simulink model "SXQCIVI"  (R2021b)
settings: Solver=FixedStepDiscrete  StartTime=0.0  StopTime=inf  FixedStep=0.005  RelTol=1e-3
undefined symbols (not defined in the file): calss, EngineTWT_Enginerunhours, EngineTWT_EnginerunhoursState, NVM_CFG_ENG_TYPE, NVM_HFV_Enginerunhours, REV_EngineSpeed, REV_EngineSpeedState, rte_set_uint32_val, rte_set_uint8_val, RXSIG_EngHrRev_Total_engine_hours, SIG_CLASS_COMTX, SIG_CLASS_NVM, SIG_CLASS_NVM_CFG, SIG_CLASS_SWC, TXSIG_EngHrRev_EGR_Total_engine_hours, TXSIG_HOURS_EGR_EngineTotalHoursofOperation, type, value
settings Model: Creator=huangyanlong  LastModifiedBy=huangyanlong
settings OptimizationCC: DefaultParameterBehavior=Inlined  EnhancedBackFolding=on  PassReuseOutputArgsAs=Individual arguments  ZeroExternalMemoryAtStartup=off  ZeroInternalMemoryAtStartup=off  OptimizeBlockOrder=speed  DifferentSizesBufferReuse=on  OptimizationCustomize=off  EfficientTunableParamExpr=on
settings DebuggingCC: ParameterTunabilityLossMsg=error
settings SFSimCC: MATLABDynamicMemAlloc=off
settings RTWCC: Description=Embedded Coder  SystemTargetFile=ert.tlc  GenCodeOnly=on  TemplateMakefile=ert_default_tmf  GenerateReport=on  IncludeHyperlinkInReport=on  LaunchReport=on  GenerateTraceInfo=on  GenerateTraceReport=on  GenerateTraceReportSl=on  GenerateTraceReportSf=on  GenerateTraceReportEml=on  GenerateWebview=on  GenerateCodeMetricsReport=on  GenerateCodeReplacementReport=on
settings CodeAppCC: ForceParamTrailComments=on  IgnoreCustomStorageClasses=off  OperatorAnnotations=on  SimulinkDataObjDesc=on  SFDataObjDesc=on  InsertBlockDesc=on
settings ERTTargetCC: TargetLangStandard=C99 (ISO)  GenerateSampleERTMain=on  InlinedParameterPlacement=NonHierarchical  ERTCustomFileTemplate=example_file_process.tlc

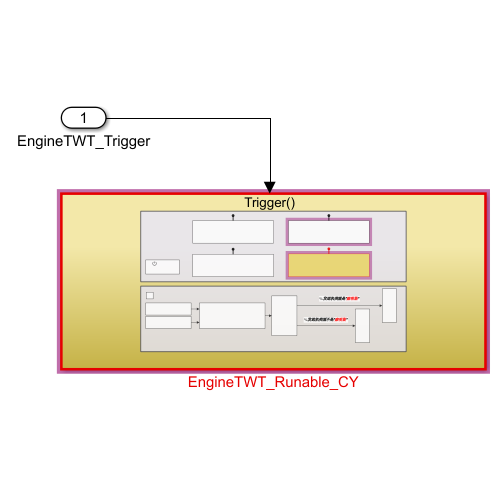
[thumbnail: Simulink's stored preview of the top-level diagram]
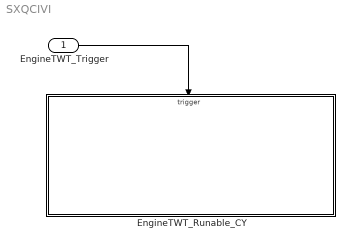
== system SXQCIVI ==
  EngineTWT_Trigger : Inport  SampleTime=0.01  OutputFunctionCall=on
  EngineTWT_Runable_CY : Subsystem
  wires:
  EngineTWT_Trigger/1 -> EngineTWT_Runable_CY/Trigger

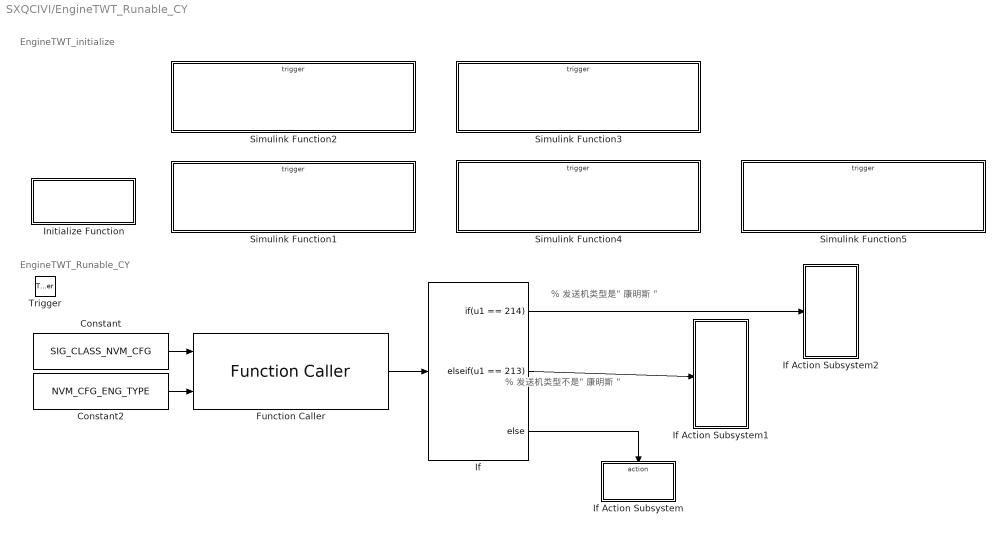
== system SXQCIVI/EngineTWT_Runable_CY ==
  note: % 发送机类型是" 康明斯 "
  note: EngineTWT_Runable_CY
  note: EngineTWT_initialize
  note: % 发送机类型不是" 康明斯 "
  Trigger : TriggerPort  TriggerType=function-call  VariantControl=(inherit)  SampleTimeType=periodic  SampleTime=0.01  PortDimensions=1
  Constant : Constant  Value=SIG_CLASS_NVM_CFG  OutDataTypeStr=int8
  Constant2 : Constant  Value=NVM_CFG_ENG_TYPE  OutDataTypeStr=int8
  Function Caller : FunctionCaller  FunctionPrototype=ret = rte_get_uint16_val(calss,type)  InputArgumentSpecifications=int8(1),int8(1)  OutputArgumentSpecifications=int16(1)
  If : If  IfExpression=u1 == 214  ElseIfExpressions=u1 == 213
  If Action Subsystem : Subsystem  TreatAsAtomicUnit=on
  If Action Subsystem1 : Subsystem  TreatAsAtomicUnit=on
  If Action Subsystem2 : Subsystem  TreatAsAtomicUnit=on
  Initialize Function : Subsystem  TreatAsAtomicUnit=on
  Simulink Function1 : Subsystem  TreatAsAtomicUnit=on
  Simulink Function2 : Subsystem  TreatAsAtomicUnit=on
  Simulink Function3 : Subsystem  TreatAsAtomicUnit=on
  Simulink Function4 : Subsystem  TreatAsAtomicUnit=on
  Simulink Function5 : Subsystem  TreatAsAtomicUnit=on
  wires:
  Constant/1 -> Function Caller/1
  Constant2/1 -> Function Caller/2
  Function Caller/1 -> If/1
  If/1 -> If Action Subsystem2/Action
  If/2 -> If Action Subsystem1/Action
  If/3 -> If Action Subsystem/Action

== system SXQCIVI/EngineTWT_Runable_CY/If Action Subsystem ==
  Action Port : ActionPort  ActionPortLabel=else

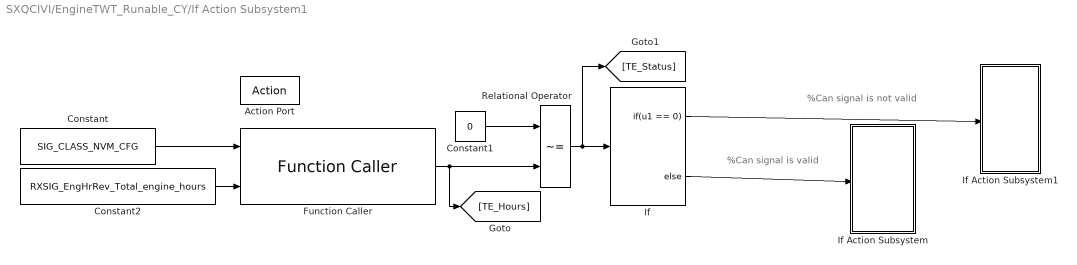
== system SXQCIVI/EngineTWT_Runable_CY/If Action Subsystem1 ==
  note: %Can signal is not valid
  note: %Can signal is valid
  Action Port : ActionPort  ActionPortLabel=elseif(u1 == 213)
  Constant : Constant  Value=SIG_CLASS_NVM_CFG  OutDataTypeStr=int8
  Constant1 : Constant  Value=0
  Constant2 : Constant  Value=RXSIG_EngHrRev_Total_engine_hours  OutDataTypeStr=int8
  Function Caller : FunctionCaller  FunctionPrototype=ret = rte_get_uint32_val(calss,type)  InputArgumentSpecifications=int8(1),int8(1)  OutputArgumentSpecifications=int32(1)
  If : If  IfExpression=u1 == 0
  If Action Subsystem : Subsystem  TreatAsAtomicUnit=on
  If Action Subsystem1 : Subsystem  TreatAsAtomicUnit=on
  Relational Operator : RelationalOperator  Operator=~=  OutDataTypeStr=boolean  RndMeth=Simplest
  wires:
  Relational Operator/1 -> [TE_Status], If/1
  Function Caller/1 -> [TE_Hours], Relational Operator/2
  Constant2/1 -> Function Caller/2
  Constant/1 -> Function Caller/1
  Constant1/1 -> Relational Operator/1
  If/1 -> If Action Subsystem1/Action
  If/2 -> If Action Subsystem/Action

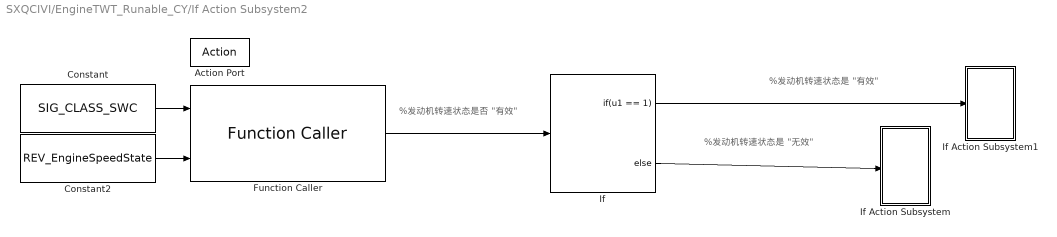
== system SXQCIVI/EngineTWT_Runable_CY/If Action Subsystem2 ==
  note: %发动机转速状态是 "有效"
  note: %发动机转速状态是否 "有效"
  note: %发动机转速状态是 "无效"
  Action Port : ActionPort  ActionPortLabel=if(u1 == 214)
  Constant : Constant  Value=SIG_CLASS_SWC  OutDataTypeStr=int8
  Constant2 : Constant  Value=REV_EngineSpeedState  OutDataTypeStr=int8
  Function Caller : FunctionCaller  FunctionPrototype=ret = rte_get_uint8_val(calss,type)  InputArgumentSpecifications=int8(1),int8(1)  OutputArgumentSpecifications=int8(1)
  If : If  IfExpression=u1 == 1
  If Action Subsystem : Subsystem  TreatAsAtomicUnit=on
  If Action Subsystem1 : Subsystem  TreatAsAtomicUnit=on
  wires:
  Constant2/1 -> Function Caller/2
  If/1 -> If Action Subsystem1/Action
  Function Caller/1 -> If/1
  Constant/1 -> Function Caller/1
  If/2 -> If Action Subsystem/Action

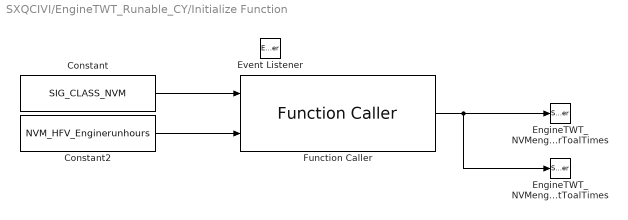
== system SXQCIVI/EngineTWT_Runable_CY/Initialize Function ==
  Constant : Constant  Value=SIG_CLASS_NVM  VectorParams1D=off  OutDataTypeStr=int8
  Constant2 : Constant  Value=NVM_HFV_Enginerunhours  OutDataTypeStr=int8
  EngineTWT_NVMengierLastToalTimes : StateWriter  StateOwnerBlock=../../If Action Subsystem2/If Action Subsystem1/Delay2  StateName=EngineTWT_NVMengierLastToalTimes
  EngineTWT_NVMengierToalTimes : StateWriter  StateOwnerBlock=../../If Action Subsystem2/If Action Subsystem1/Delay1  StateName=EngineTWT_NVMengierToalTimes
  Event Listener : EventListener  DisableCoverage=on  EventName=reset
  Function Caller : FunctionCaller  FunctionPrototype=ret = rte_get_uint32_val(calss,type)  InputArgumentSpecifications=int8(1),int8(1)  OutputArgumentSpecifications=int32(1)
  wires:
  Constant/1 -> Function Caller/1
  Constant2/1 -> Function Caller/2
  Function Caller/1 -> EngineTWT_NVMengierLastToalTimes/1, EngineTWT_NVMengierToalTimes/1

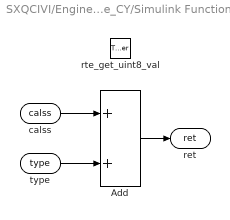
== system SXQCIVI/EngineTWT_Runable_CY/Simulink Function1 ==
  rte_get_uint8_val : TriggerPort  TriggerType=function-call  IsSimulinkFunction=on  FunctionName=rte_get_uint8_val  FunctionVisibility=scoped  VariantControl=(inherit)
  Add : Sum
  calss : ArgIn  DisableCoverage=on  OutDataTypeStr=int8  ArgumentName=calss
  type : ArgIn  Port=2  OutDataTypeStr=int8  ArgumentName=type
  ret : ArgOut  DisableCoverage=on  OutDataTypeStr=int8  ArgumentName=ret
  wires:
  Add/1 -> ret/1
  type/1 -> Add/2
  calss/1 -> Add/1

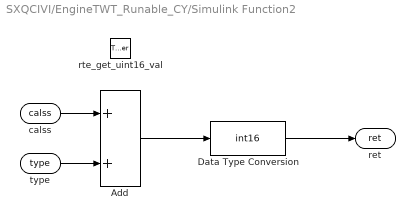
== system SXQCIVI/EngineTWT_Runable_CY/Simulink Function2 ==
  rte_get_uint16_val : TriggerPort  TriggerType=function-call  IsSimulinkFunction=on  FunctionName=rte_get_uint16_val  FunctionVisibility=scoped  VariantControl=(inherit)
  Add : Sum
  Data Type Conversion : DataTypeConversion  OutDataTypeStr=int16
  calss : ArgIn  DisableCoverage=on  OutDataTypeStr=int8  ArgumentName=calss
  type : ArgIn  Port=2  OutDataTypeStr=int8  ArgumentName=type
  ret : ArgOut  DisableCoverage=on  OutDataTypeStr=int16  ArgumentName=ret
  wires:
  calss/1 -> Add/1
  type/1 -> Add/2
  Add/1 -> Data Type Conversion/1
  Data Type Conversion/1 -> ret/1

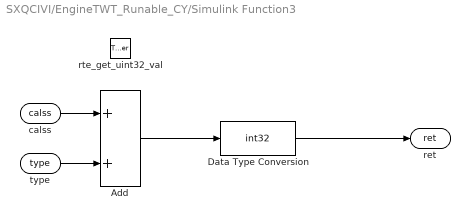
== system SXQCIVI/EngineTWT_Runable_CY/Simulink Function3 ==
  rte_get_uint32_val : TriggerPort  TriggerType=function-call  IsSimulinkFunction=on  FunctionName=rte_get_uint32_val  FunctionVisibility=scoped  VariantControl=(inherit)
  Add : Sum
  Data Type Conversion : DataTypeConversion  OutDataTypeStr=int32
  calss : ArgIn  DisableCoverage=on  OutDataTypeStr=int8  ArgumentName=calss
  type : ArgIn  Port=2  OutDataTypeStr=int8  ArgumentName=type
  ret : ArgOut  DisableCoverage=on  OutDataTypeStr=int32  ArgumentName=ret
  wires:
  Add/1 -> Data Type Conversion/1
  type/1 -> Add/2
  calss/1 -> Add/1
  Data Type Conversion/1 -> ret/1

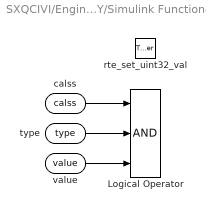
== system SXQCIVI/EngineTWT_Runable_CY/Simulink Function4 ==
  rte_set_uint32_val : TriggerPort  TriggerType=function-call  IsSimulinkFunction=on  FunctionName=rte_set_uint32_val  FunctionVisibility=scoped  VariantControl=(inherit)
  Logical Operator : Logic  Inputs=3  AllPortsSameDT=off  OutDataTypeStr=boolean
  calss : ArgIn  DisableCoverage=on  OutDataTypeStr=int8  ArgumentName=calss
  type : ArgIn  Port=2  OutDataTypeStr=int16  ArgumentName=type
  value : ArgIn  Port=3  OutDataTypeStr=int32  ArgumentName=value
  wires:
  calss/1 -> Logical Operator/1
  type/1 -> Logical Operator/2
  value/1 -> Logical Operator/3

== system SXQCIVI/EngineTWT_Runable_CY/Simulink Function5 ==
  rte_set_uint8_val : TriggerPort  TriggerType=function-call  IsSimulinkFunction=on  FunctionName=rte_set_uint8_val  FunctionVisibility=scoped  VariantControl=(inherit)
  Logical Operator : Logic  Inputs=3  AllPortsSameDT=off  OutDataTypeStr=boolean
  calss : ArgIn  DisableCoverage=on  OutDataTypeStr=int8  ArgumentName=calss
  type : ArgIn  Port=2  OutDataTypeStr=int16  ArgumentName=type
  value : ArgIn  Port=3  OutDataTypeStr=int8  ArgumentName=value
  wires:
  value/1 -> Logical Operator/3
  type/1 -> Logical Operator/2
  calss/1 -> Logical Operator/1

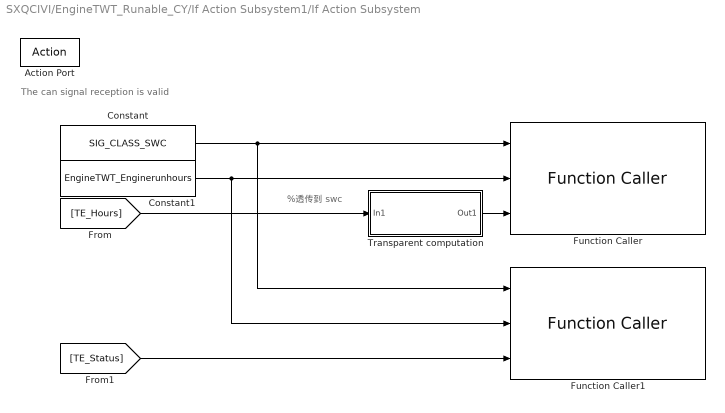
== system SXQCIVI/EngineTWT_Runable_CY/If Action Subsystem1/If Action Subsystem ==
  note: The can signal reception is valid
  note: %透传到 swc
  Action Port : ActionPort  ActionPortLabel=else
  Constant : Constant  Value=SIG_CLASS_SWC  OutDataTypeStr=int8
  Constant1 : Constant  Value=EngineTWT_Enginerunhours  OutDataTypeStr=int16
  Function Caller : FunctionCaller  FunctionPrototype=rte_set_uint32_val(calss,type,value)  InputArgumentSpecifications=int8(1),int16(1),int32(1)
  Function Caller1 : FunctionCaller  FunctionPrototype=rte_set_uint32_val(calss,type,value)  InputArgumentSpecifications=int8(1),int16(1),int32(1)
  Transparent computation : Subsystem
  wires:
  Constant1/1 -> Function Caller1/2, Function Caller/2
  [TE_Status] -> Function Caller1/3
  [TE_Hours] -> Transparent computation/1(In1)
  Transparent computation/1(Out1) -> Function Caller/3
  Constant/1 -> Function Caller1/1, Function Caller/1

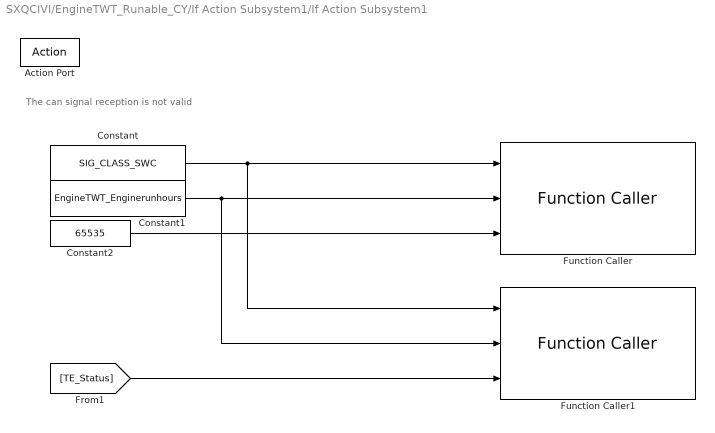
== system SXQCIVI/EngineTWT_Runable_CY/If Action Subsystem1/If Action Subsystem1 ==
  note: The can signal reception is not valid
  Action Port : ActionPort  ActionPortLabel=if(u1 == 0)
  Constant : Constant  Value=SIG_CLASS_SWC  OutDataTypeStr=int8
  Constant1 : Constant  Value=EngineTWT_Enginerunhours  OutDataTypeStr=int16
  Constant2 : Constant  Value=65535  OutDataTypeStr=int32
  Function Caller : FunctionCaller  FunctionPrototype=rte_set_uint32_val(calss,type,value)  InputArgumentSpecifications=int8(1),int16(1),int32(1)
  Function Caller1 : FunctionCaller  FunctionPrototype=rte_set_uint8_val(calss,type,value)  InputArgumentSpecifications=int8(1),int16(1),int8(1)
  wires:
  Constant2/1 -> Function Caller/3
  Constant/1 -> Function Caller1/1, Function Caller/1
  Constant1/1 -> Function Caller1/2, Function Caller/2
  [TE_Status] -> Function Caller1/3

== system SXQCIVI/EngineTWT_Runable_CY/If Action Subsystem2/If Action Subsystem ==
  note: The Engine speed effective
  Action Port : ActionPort  ActionPortLabel=else

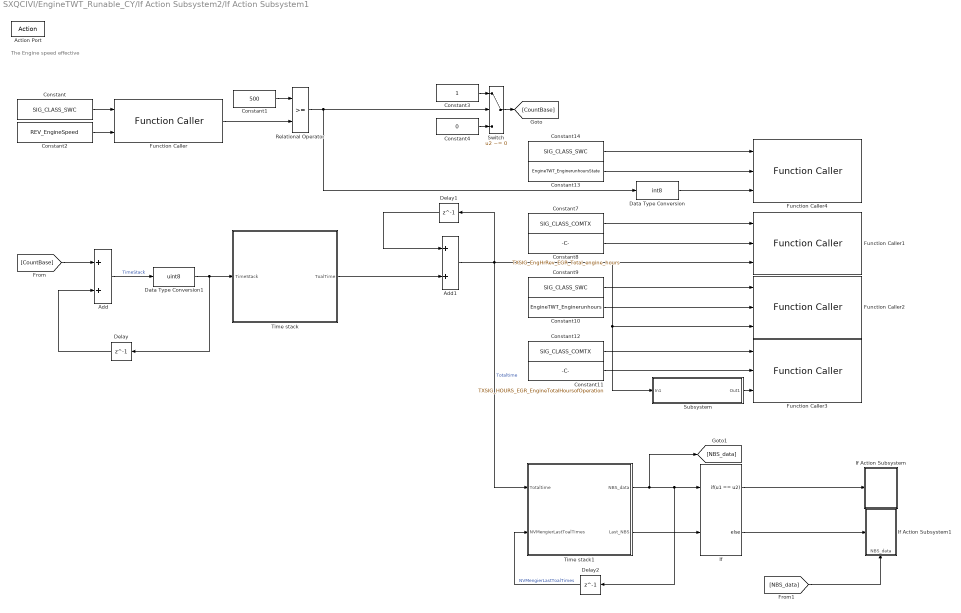
== system SXQCIVI/EngineTWT_Runable_CY/If Action Subsystem2/If Action Subsystem1 ==
  note: The Engine speed effective
  Action Port : ActionPort  ActionPortLabel=if(u1 == 1)
  Add : Sum
  Add1 : Sum
  Constant : Constant  Value=SIG_CLASS_SWC  OutDataTypeStr=int8
  Constant1 : Constant  Value=500
  Constant10 : Constant  Value=EngineTWT_Enginerunhours  OutDataTypeStr=int16
  Constant11 : Constant  Value=TXSIG_HOURS_EGR_EngineTotalHoursofOperation  OutDataTypeStr=int16
  Constant12 : Constant  Value=SIG_CLASS_COMTX  OutDataTypeStr=int8
  Constant13 : Constant  Value=EngineTWT_EnginerunhoursState  OutDataTypeStr=int16
  Constant14 : Constant  Value=SIG_CLASS_SWC  OutDataTypeStr=int8
  Constant2 : Constant  Value=REV_EngineSpeed  OutDataTypeStr=int8
  Constant3 : Constant
  Constant4 : Constant  Value=0
  Constant7 : Constant  Value=SIG_CLASS_COMTX  OutDataTypeStr=int8
  Constant8 : Constant  Value=TXSIG_EngHrRev_EGR_Total_engine_hours  OutDataTypeStr=int16
  Constant9 : Constant  Value=SIG_CLASS_SWC  OutDataTypeStr=int8
  Data Type Conversion : DataTypeConversion  OutDataTypeStr=int8
  Data Type Conversion1 : DataTypeConversion  OutDataTypeStr=uint8
  Delay : Delay  DelayLength=1
  Delay1 : Delay  DelayLength=1  StateName=EngineTWT_NVMengierToalTimes
  Delay2 : Delay  DelayLength=1  StateName=EngineTWT_NVMengierLastToalTimes  StateMustResolveToSignalObject=on
  Function Caller : FunctionCaller  FunctionPrototype=ret = rte_get_uint16_val(calss,type)  InputArgumentSpecifications=int8(1),int8(1)  OutputArgumentSpecifications=int16(1)
  Function Caller1 : FunctionCaller  FunctionPrototype=rte_set_uint32_val(calss,type,value)  InputArgumentSpecifications=int8(1),int16(1),int32(1)
  Function Caller2 : FunctionCaller  FunctionPrototype=rte_set_uint32_val(calss,type,value)  InputArgumentSpecifications=int8(1),int16(1),int32(1)
  Function Caller3 : FunctionCaller  FunctionPrototype=rte_set_uint32_val(calss,type,value)  InputArgumentSpecifications=int8(1),int16(1),int32(1)
  Function Caller4 : FunctionCaller  FunctionPrototype=rte_set_uint8_val(calss,type,value)  InputArgumentSpecifications=int8(1),int16(1),int8(1)
  If : If  NumInputs=2  IfExpression=u1 == u2
  If Action Subsystem : Subsystem  TreatAsAtomicUnit=on
  If Action Subsystem1 : Subsystem  TreatAsAtomicUnit=on
  Relational Operator : RelationalOperator  OutDataTypeStr=boolean  RndMeth=Simplest
  Subsystem : Subsystem
  Switch : Switch  Criteria=u2 ~= 0
  Time stack : Stateflow chart  TreatAsAtomicUnit=on
  Time stack1 : Stateflow chart  TreatAsAtomicUnit=on
  wires:
  Constant8/1 -> Function Caller1/2
  [CountBase] -> Add/1
  Switch/1 -> [CountBase]
  Constant/1 -> Function Caller/1
  Constant4/1 -> Switch/3
  Subsystem/1(Out1) -> Function Caller3/3
  Time stack1/1(NBS_data) -> [NBS_data], Delay2/1, If/1
  Constant2/1 -> Function Caller/2
  Constant3/1 -> Switch/1
  Delay2/1 -> Time stack1/2(NVMengierLastToalTimes)  "NVMengierLastToalTimes"
  If/2 -> If Action Subsystem1/Action
  Time stack/1(ToalTime) -> Add1/2
  If/1 -> If Action Subsystem/Action
  Constant13/1 -> Function Caller4/2
  Constant14/1 -> Function Caller4/1
  Relational Operator/1 -> Data Type Conversion/1, Switch/2
  Delay/1 -> Add/2
  Constant1/1 -> Relational Operator/1
  Add/1 -> Data Type Conversion1/1  "TimeStack"
  [NBS_data] -> If Action Subsystem1/1(NBS_data)
  Time stack1/2(Last_NBS) -> If/2
  Delay1/1 -> Add1/1
  Constant10/1 -> Function Caller2/2
  Constant12/1 -> Function Caller3/1
  Add1/1 -> Time stack1/1(Totaltime), Delay1/1, Subsystem/1(In1), Function Caller2/3, Function Caller1/3  "Totaltime"
  Constant11/1 -> Function Caller3/2
  Constant7/1 -> Function Caller1/1
  Constant9/1 -> Function Caller2/1
  Function Caller/1 -> Relational Operator/2
  Data Type Conversion/1 -> Function Caller4/3
  Data Type Conversion1/1 -> Delay/1, Time stack/1(TimeStack)

== system SXQCIVI/EngineTWT_Runable_CY/If Action Subsystem1/If Action Subsystem/Transparent computation ==
  In1 : Inport
  Gain : Gain  Gain=0.5  ParamDataTypeStr=int32  OutDataTypeStr=int32
  Out1 : Outport
  wires:
  In1/1 -> Gain/1
  Gain/1 -> Out1/1

== system SXQCIVI/EngineTWT_Runable_CY/If Action Subsystem2/If Action Subsystem1/If Action Subsystem ==
  Action Port : ActionPort  ActionPortLabel=if(u1 == u2)

== system SXQCIVI/EngineTWT_Runable_CY/If Action Subsystem2/If Action Subsystem1/If Action Subsystem1 ==
  NBS_data : Inport
  Action Port : ActionPort  ActionPortLabel=else
  Constant5 : Constant  Value=NVM_HFV_Enginerunhours  OutDataTypeStr=int16
  Constant6 : Constant  Value=SIG_CLASS_NVM  OutDataTypeStr=int8
  Function Caller5 : FunctionCaller  FunctionPrototype=rte_set_uint32_val(calss,type,value)  InputArgumentSpecifications=int8(1),int16(1),int32(1)
  wires:
  NBS_data/1 -> Function Caller5/3
  Constant5/1 -> Function Caller5/2
  Constant6/1 -> Function Caller5/1

== system SXQCIVI/EngineTWT_Runable_CY/If Action Subsystem2/If Action Subsystem1/Subsystem ==
  In1 : Inport
  Gain : Gain  Gain=2  OutDataTypeStr=int32
  Out1 : Outport
  wires:
  In1/1 -> Gain/1
  Gain/1 -> Out1/1

== stateflow chart SXQCIVI/EngineTWT_Runable_CY/If Action Subsystem2/If Action Subsystem1/Time stack ==
  state IDLE
    entry:  ToalTime = 0x00;
    during:ToalTime  =0x00;
  state Add
    entry:  ToalTime = 0x01;Local_Time  =TimeStack;
    during:ToalTime = 0x01;Local_Time  =TimeStack;
  (default) -> IDLE : {Local_Time = 0x00;}
  IDLE -> Add : [(TimeStack - Local_Time) == 6000 ]
  Add -> IDLE : {ToalTime == 0x00;}
  data: TimeStack input uint8; ToalTime output; Local_Time local uint8

== stateflow chart SXQCIVI/EngineTWT_Runable_CY/If Action Subsystem2/If Action Subsystem1/Time stack1 ==
  state IDLE
    during:TimeCnt = TimeCnt+1;
  state start
    entry:NBS_data = Totaltime;
  (default) -> IDLE : {NBS_data = NVMengierLastToalTimes;
      | Last_NBS = NVMengierLastToalTimes;}
  IDLE -> start : [TimeCnt == 5400]
  start -> IDLE : {TimeCnt = 0;}
  data: TimeCnt local; Totaltime input; NBS_data output; NVMengierLastToalTimes input; Last_NBS output
